simulink model "AUV_Model"  (Simulink 8.2)
settings: Solver=ode4  StartTime=0.0  StopTime=20  FixedStep=0.1  RelTol=1e-3
model workspace (MAT data in the model file):
  cg = Simulink.Signal
  cg.DataType = 'double'
  cg.DocUnits = 'm'
  cg.Dimensions = 3
  cg.DimensionsMode = 'auto'
  cg.Complexity = 'real'
  cg.SampleTime = -1
  cg.SamplingMode = 'Sample based'
  cg.InitialValue = '[0 0 0]'
  m = Simulink.Signal
  m.DataType = 'double'
  m.DocUnits = 'kg'
  m.Dimensions = 1
  m.DimensionsMode = 'auto'
  m.Complexity = 'real'
  m.SampleTime = -1
  m.SamplingMode = 'auto'
  m.InitialValue = '39.00'
  L = Simulink.Signal
  L.DataType = 'double'
  L.DocUnits = 'm'
  L.Dimensions = 1
  L.DimensionsMode = 'auto'
  L.Complexity = 'real'
  L.SampleTime = -1
  L.SamplingMode = 'auto'
  L.InitialValue = '1.065'
  rho = Simulink.Signal
  rho.DataType = 'double'
  rho.DocUnits = 'Kg/m3'
  rho.Dimensions = 1
  rho.DimensionsMode = 'auto'
  rho.Complexity = 'real'
  rho.SampleTime = -1
  rho.SamplingMode = 'auto'
  rho.InitialValue = '1000'
  R = Simulink.Signal
  R.DataType = 'double'
  R.DocUnits = 'm'
  R.Dimensions = 1
  R.DimensionsMode = 'auto'
  R.Complexity = 'real'
  R.SampleTime = -1
  R.SamplingMode = 'auto'
  R.InitialValue = '0.125'
  cb = Simulink.Signal
  cb.DataType = 'double'
  cb.DocUnits = 'm'
  cb.Dimensions = 3
  cb.DimensionsMode = 'auto'
  cb.Complexity = 'real'
  cb.SampleTime = -1
  cb.SamplingMode = 'auto'
  cb.InitialValue = '[0 0 0]'
PostLoadFcn:
  | , if any(exist('dsrtsu_mdlpostloadfcn', 'file') == [2, 3, 6]), try dsrtsu_mdlpostloadfcn('Execute', bdroot); catch fprintf('Error in PostLoadFcn (dsrtsu_mdlpostloadfcn) for model "%s":\n %s\n', bdroot, lasterr); end, end,
InitFcn:
  | b=0;
  | xi=10;
  | yi=10;
  | zi=10;
  | Yawi =0;
  | 
  | x=xi;
  | y=yi;
  | z=zi;
  | yaw=Yawi;
  | pitch=0;
  | roll=0;
  | 
  | xf=20
  | yf=20
  | zf=10
  | %desired time to destination
  | Tdes = 20;
  | 
  | %step count
  | n=Tdes/0.100
StopFcn:
  | % plot3(x,y,-z)
  | plot(x,y)
  |  grid on
  |  axis square
  |  xlabel('x,Surge')
  |  ylabel('y,Sway')
  | % zlabel('-z,Heave')
  |  title('Plot of the AUV path','FontSize',12)
  | % set(p,'Color','red','LineWidth',1)
undefined symbols (not defined in the file): kix, kiy, kpx, kpy
settings Model: DSRTSU_INTERNAL_RTI_VER=360  DSRTSU_INTERNAL_RTI_TYPE=rti1104  Creator=Umesh  LastModifiedBy=Dr. Asokan  ModifiedComment=Umesh -- Fri Jul 22 10:55:36 2011 -- Version 1.4
settings Model: ModifiedHistory=|
  | Umesh -- Fri Jul 22 10:55:36 2011 -- Version 1.4
  | 
  | 
  | Umesh -- Fri Jul 22 10:53:33 2011 -- Version 1.3
  | 
  | 
  | Umesh -- Fri Jul 22 10:49:07 2011 -- Version 1.2
  | 
  | 
  | Umesh -- Fri Jul 22 01:17:32 2011 -- Version 1.1
  | Initial Version of a simple cylindrically shaped AUV
settings OptimizationCC: SimCompilerOptimization=On
settings HardwareCC: ProdIntDivRoundTo=Zero  ProdEndianess=BigEndian  ProdHWDeviceType=Generic->Custom  TargetIntDivRoundTo=Zero  TargetEndianess=BigEndian  TargetHWDeviceType=Generic->Custom
settings SFSimCC: SimParseCustomCode=off
settings RTWCC: SystemTargetFile=rti1104.tlc  MakeCommand=make_rti  TemplateMakefile=rti1104.tmf  Description=dSPACE DS1104 Hardware Platform  ProcessScript=rti1104_make_rtw_hook
settings STFCustomTargetCC: CodeReplacementLibrary=ANSI_C  ParMdlRefBuildCompliant=on  GeneratePreprocessorConditionals=Disable all  SystemTargetFile=rti1104.tlc
settings GRTTargetCC: CompOptLevelCompliant=off  ConcurrentExecutionCompliant=off  MatFileLogging=off  ExtModeMexFile=noextcomm
settings CustomProperty: DataType=RTWOptions_EnumType_F__Installed_Soft_dSPACE_6P6_matlab_rti1104_tlc_rti1104_1InitialSimState  Value=RUN
settings EnumStrPairs: String=RUN

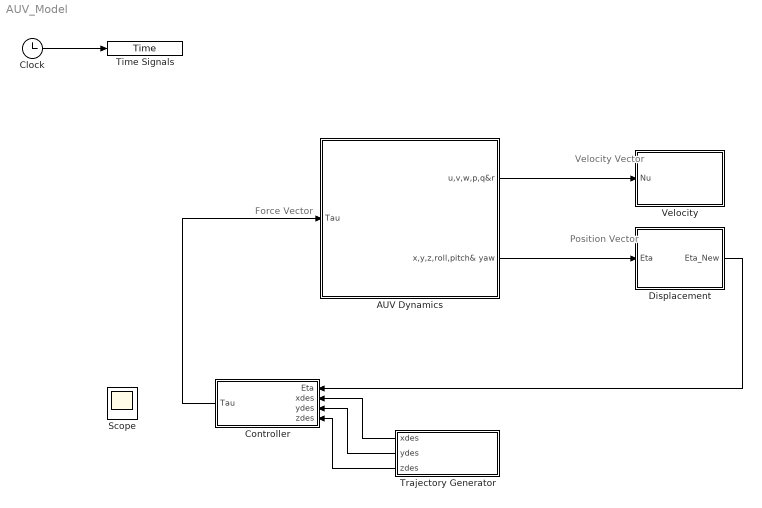
== system AUV_Model ==
  note: Position Vector
  note: Velocity Vector
  note: Force Vector
  AUV Dynamics : Subsystem  Description=Modelled Dynamics of Jubilee AUV, developed by Robotics Lab, IIT Madras
      mask Display: image(imread('Jubilee.jpg'))
  Clock : Clock
  Controller : Subsystem
  Displacement : Subsystem
  Scope : Scope
  Time Signals : ToWorkspace  VariableName=Time  SampleTime=-1
  Trajectory Generator : Subsystem
  Velocity : Subsystem
  wires:
  Clock/1 -> Time Signals/1
  AUV Dynamics/2(x,y,z,roll,pitch& yaw) -> Displacement/1(Eta)
  AUV Dynamics/1(u,v,w,p,q&r) -> Velocity/1(Nu)
  Displacement/1(Eta_New) -> Controller/1(Eta)
  Controller/1(Tau) -> AUV Dynamics/1(Tau)
  Trajectory Generator/2(ydes) -> Controller/3(ydes)
  Trajectory Generator/3(zdes) -> Controller/4(zdes)
  Trajectory Generator/1(xdes) -> Controller/2(xdes)

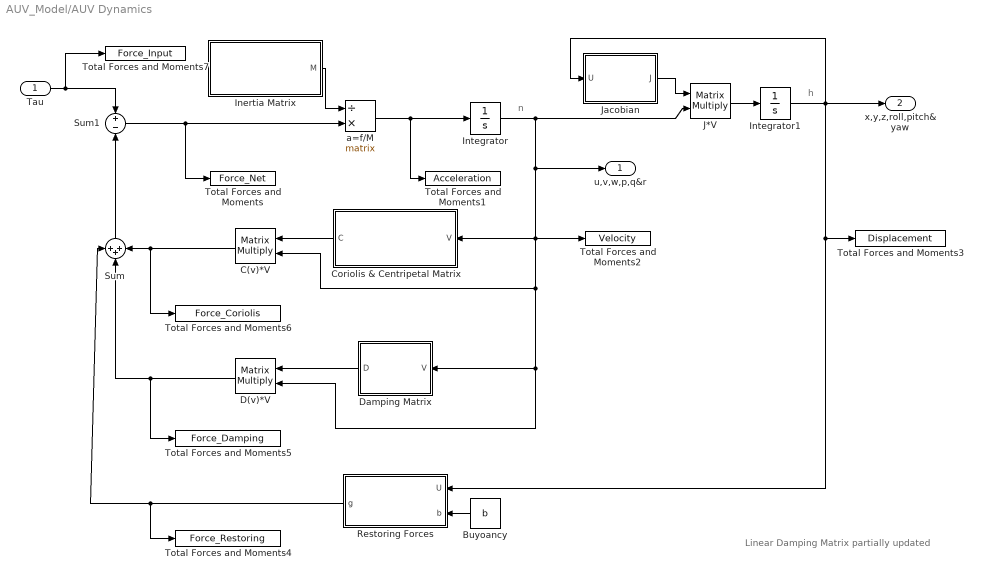
== system AUV_Model/AUV Dynamics ==
  note: h
  note: n
  note: Linear Damping Matrix partially updated
  Tau : Inport
  Buyoancy : Constant  Value=b
  C(v)*V : Product  Inputs=**  Multiplication=Matrix(*)
  Coriolis & Centripetal Matrix : MATLAB Function  TreatAsAtomicUnit=on
  D(v)*V : Product  Inputs=**  Multiplication=Matrix(*)
  Damping Matrix : MATLAB Function  TreatAsAtomicUnit=on
  Inertia Matrix : MATLAB Function  Description=Sub program for Inertia and added mass matrix  TreatAsAtomicUnit=on
  Integrator : Integrator  InitialCondition=[0 0 0 0 0 0]'
  Integrator1 : Integrator  InitialCondition=[xi yi zi 0 0 Yawi*pi/180]'
  J*V : Product  Inputs=**  Multiplication=Matrix(*)
  Jacobian : MATLAB Function  TreatAsAtomicUnit=on
  Restoring Forces : MATLAB Function  TreatAsAtomicUnit=on
  Sum : Sum  Inputs=+++
  Sum1 : Sum  Inputs=+-
  Total Forces and Moments : ToWorkspace  VariableName=Force_Net  SampleTime=-1
  Total Forces and Moments1 : ToWorkspace  VariableName=Acceleration  SampleTime=-1
  Total Forces and Moments2 : ToWorkspace  VariableName=Velocity  SampleTime=-1
  Total Forces and Moments3 : ToWorkspace  VariableName=Displacement  SampleTime=-1
  Total Forces and Moments4 : ToWorkspace  VariableName=Force_Restoring  SampleTime=-1
  Total Forces and Moments5 : ToWorkspace  VariableName=Force_Damping  SampleTime=-1
  Total Forces and Moments6 : ToWorkspace  VariableName=Force_Coriolis  SampleTime=-1
  Total Forces and Moments7 : ToWorkspace  VariableName=Force_Input  SampleTime=-1
  a=f/M : Product  Inputs=/*  Multiplication=Matrix(*)
  u,v,w,p,q&r : Outport
  x,y,z,roll,pitch& yaw : Outport  Port=2
  wires:
  Tau/1 -> Sum1/1, Total Forces and Moments7/1
  Sum1/1 -> Total Forces and Moments/1, a=f/M/2
  a=f/M/1 -> Total Forces and Moments1/1, Integrator/1
  Integrator/1 -> J*V/2, Total Forces and Moments2/1, Coriolis & Centripetal Matrix/1(V), C(v)*V/2, D(v)*V/2, Damping Matrix/1(V), u,v,w,p,q&r/1
  J*V/1 -> Integrator1/1
  Buyoancy/1 -> Restoring Forces/2(b)
  Restoring Forces/1(g) -> Sum/1, Total Forces and Moments4/1
  Sum/1 -> Sum1/2
  D(v)*V/1 -> Sum/2, Total Forces and Moments5/1
  C(v)*V/1 -> Sum/3, Total Forces and Moments6/1
  Integrator1/1 -> x,y,z,roll,pitch& yaw/1, Restoring Forces/1(U), Total Forces and Moments3/1, Jacobian/1(U)
  Jacobian/1(J) -> J*V/1
  Damping Matrix/1(D) -> D(v)*V/1
  Coriolis & Centripetal Matrix/1(C) -> C(v)*V/1
  Inertia Matrix/1(M) -> a=f/M/1

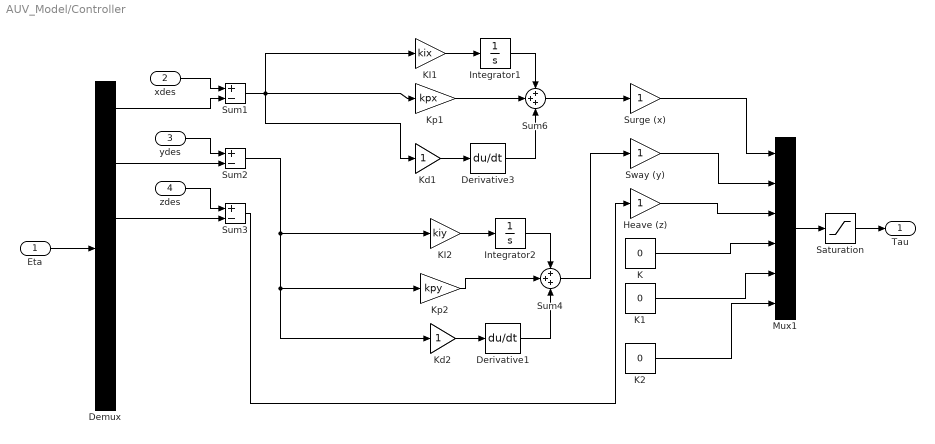
== system AUV_Model/Controller ==
  Eta : Inport
  xdes : Inport  Port=2
  ydes : Inport  Port=3
  zdes : Inport  Port=4
  Demux : Demux  Outputs=6
  Derivative1 : Derivative
  Derivative3 : Derivative
  Heave (z) : Gain
  Integrator1 : Integrator
  Integrator2 : Integrator
  K : Constant  Value=0
  K1 : Constant  Value=0
  K2 : Constant  Value=0
  KI1 : Gain  Gain=kix
  KI2 : Gain  Gain=kiy
  Kd1 : Gain
  Kd2 : Gain
  Kp1 : Gain  Gain=kpx
  Kp2 : Gain  Gain=kpy
  Mux1 : Mux  Inputs=6
  Saturation : Saturate  UpperLimit=56.9  LowerLimit=-56.9
  Sum1 : Sum  Inputs=+-
  Sum2 : Sum  Inputs=+-
  Sum3 : Sum  Inputs=+-
  Sum4 : Sum  Inputs=+++
  Sum6 : Sum  Inputs=+++
  Surge (x) : Gain
  Sway (y) : Gain
  Tau : Outport
  wires:
  Eta/1 -> Demux/1
  xdes/1 -> Sum1/1
  ydes/1 -> Sum2/1
  zdes/1 -> Sum3/1
  Mux1/1 -> Saturation/1
  Sum1/1 -> Kp1/1, KI1/1, Kd1/1
  Sum2/1 -> Kp2/1, Kd2/1, KI2/1
  Sum3/1 -> Heave (z)/1
  Surge (x)/1 -> Mux1/1
  Sway (y)/1 -> Mux1/2
  Heave (z)/1 -> Mux1/3
  K/1 -> Mux1/4
  K1/1 -> Mux1/5
  K2/1 -> Mux1/6
  Saturation/1 -> Tau/1
  Demux/1 -> Sum1/2
  Demux/2 -> Sum2/2
  Demux/3 -> Sum3/2
  Kd1/1 -> Derivative3/1
  KI1/1 -> Integrator1/1
  Integrator1/1 -> Sum6/1
  Derivative3/1 -> Sum6/3
  Kp1/1 -> Sum6/2
  Sum6/1 -> Surge (x)/1
  Kd2/1 -> Derivative1/1
  KI2/1 -> Integrator2/1
  Integrator2/1 -> Sum4/1
  Derivative1/1 -> Sum4/3
  Kp2/1 -> Sum4/2
  Sum4/1 -> Sway (y)/1

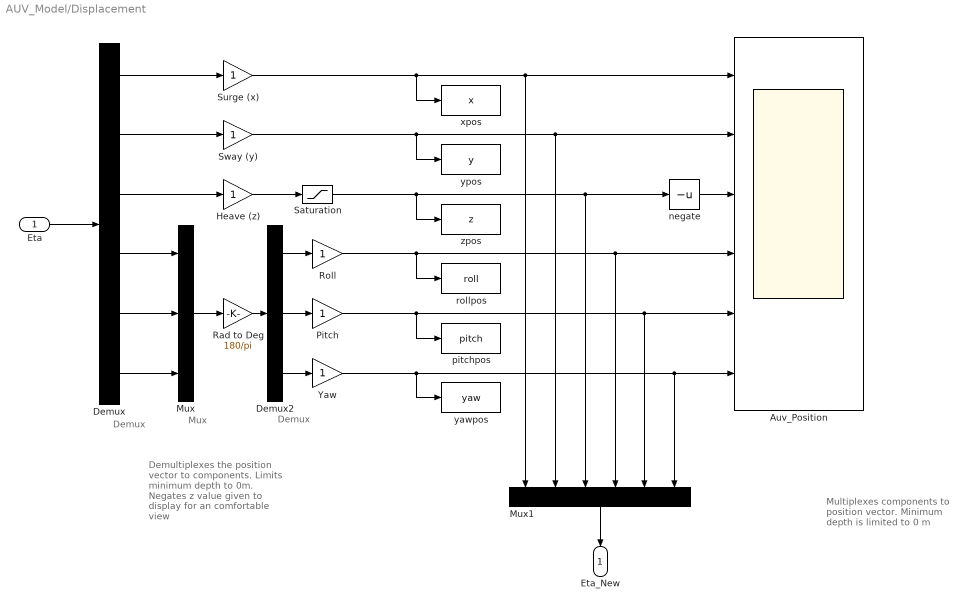
== system AUV_Model/Displacement ==
  note: Demux
  note: Mux
  note: Demux
  note: Demultiplexes the position vector to components.
      | Limits minimum depth to 0m.
      | Negates z value given to display for an comfortable view
  note: Multiplexes components to position vector.
      | Minimum depth is limited to 0 m
  Eta : Inport
  Auv_Position : Scope  NumInputPorts=6
      settings: TickLabels=on  YMin=-50~-1~-25~-1~0~-1  YMax=0~1~-0~1~4~1  SaveName=ScopeData24  MaxDataPoints=10000
  Demux : Demux  Outputs=6
  Demux2 : Demux  Outputs=3
  Heave (z) : Gain
  Mux : Mux  Inputs=3
  Mux1 : Mux  Inputs=6
  Pitch : Gain
  Rad to Deg : Gain  Gain=180/pi
  Roll : Gain
  Saturation : Saturate  UpperLimit=inf  LowerLimit=0
  Surge (x) : Gain
  Sway (y) : Gain
  Yaw : Gain
  negate : UnaryMinus
  pitchpos : ToWorkspace  VariableName=pitch  SampleTime=-1
  rollpos : ToWorkspace  VariableName=roll  SampleTime=-1
  xpos : ToWorkspace  VariableName=x  SampleTime=-1
  yawpos : ToWorkspace  VariableName=yaw  SampleTime=-1
  ypos : ToWorkspace  VariableName=y  SampleTime=-1
  zpos : ToWorkspace  VariableName=z  SampleTime=-1
  Eta_New : Outport
  wires:
  Demux2/3 -> Yaw/1
  Demux2/2 -> Pitch/1
  Demux2/1 -> Roll/1
  Demux/3 -> Heave (z)/1
  Demux/2 -> Sway (y)/1
  Demux/1 -> Surge (x)/1
  Rad to Deg/1 -> Demux2/1
  Mux/1 -> Rad to Deg/1
  Demux/4 -> Mux/1
  Demux/6 -> Mux/3
  Demux/5 -> Mux/2
  Eta/1 -> Demux/1
  Surge (x)/1 -> xpos/1, Auv_Position/1, Mux1/1
  Sway (y)/1 -> ypos/1, Auv_Position/2, Mux1/2
  Heave (z)/1 -> Saturation/1
  negate/1 -> Auv_Position/3
  Saturation/1 -> zpos/1, negate/1, Mux1/3
  Roll/1 -> rollpos/1, Auv_Position/4, Mux1/4
  Pitch/1 -> pitchpos/1, Auv_Position/5, Mux1/5
  Yaw/1 -> yawpos/1, Auv_Position/6, Mux1/6
  Mux1/1 -> Eta_New/1

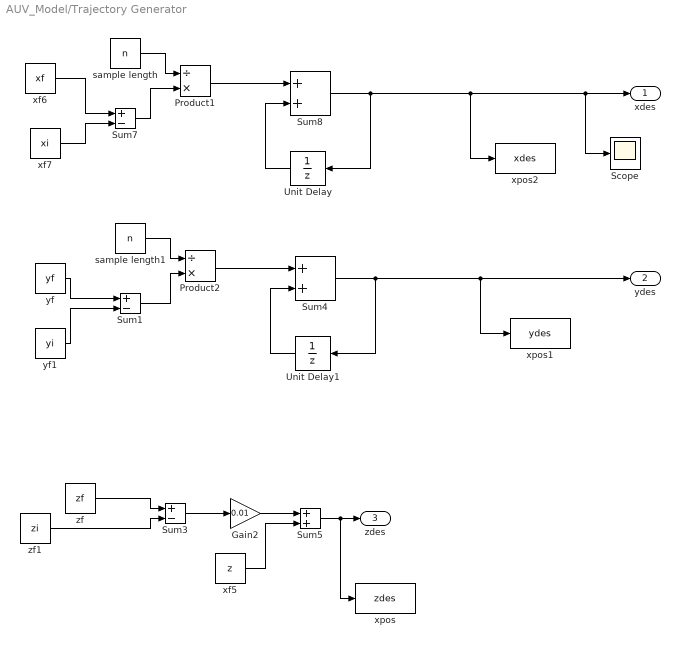
== system AUV_Model/Trajectory Generator ==
  Gain2 : Gain  Gain=0.01
  Product1 : Product  Inputs=/*  RndMeth=Zero
  Product2 : Product  Inputs=/*  RndMeth=Zero
  Scope : Scope
  Sum1 : Sum  Inputs=+-
  Sum3 : Sum  Inputs=+-
  Sum4 : Sum
  Sum5 : Sum
  Sum7 : Sum  Inputs=+-
  Sum8 : Sum
  Unit Delay : UnitDelay  SampleTime=-1
  Unit Delay1 : UnitDelay  SampleTime=-1
  sample length : Constant  Value=n
  sample length1 : Constant  Value=n
  xf5 : Constant  Value=z
  xf6 : Constant  Value=xf
  xf7 : Constant  Value=xi
  xpos : ToWorkspace  VariableName=zdes  SampleTime=-1
  xpos1 : ToWorkspace  VariableName=ydes  SampleTime=-1
  xpos2 : ToWorkspace  VariableName=xdes  SampleTime=-1
  yf : Constant  Value=yf
  yf1 : Constant  Value=yi
  zf : Constant  Value=zf
  zf1 : Constant  Value=zi
  xdes : Outport
  ydes : Outport  Port=2
  zdes : Outport  Port=3
  wires:
  zf1/1 -> Sum3/2
  zf/1 -> Sum3/1
  Sum3/1 -> Gain2/1
  Gain2/1 -> Sum5/1
  Sum5/1 -> zdes/1, xpos/1
  xf5/1 -> Sum5/2
  xf7/1 -> Sum7/2
  xf6/1 -> Sum7/1
  Sum7/1 -> Product1/2
  sample length/1 -> Product1/1
  Product1/1 -> Sum8/1
  Sum8/1 -> Unit Delay/1, Scope/1, xdes/1, xpos2/1
  Unit Delay/1 -> Sum8/2
  Sum1/1 -> Product2/2
  sample length1/1 -> Product2/1
  Product2/1 -> Sum4/1
  Sum4/1 -> Unit Delay1/1, ydes/1, xpos1/1
  Unit Delay1/1 -> Sum4/2
  yf1/1 -> Sum1/2
  yf/1 -> Sum1/1

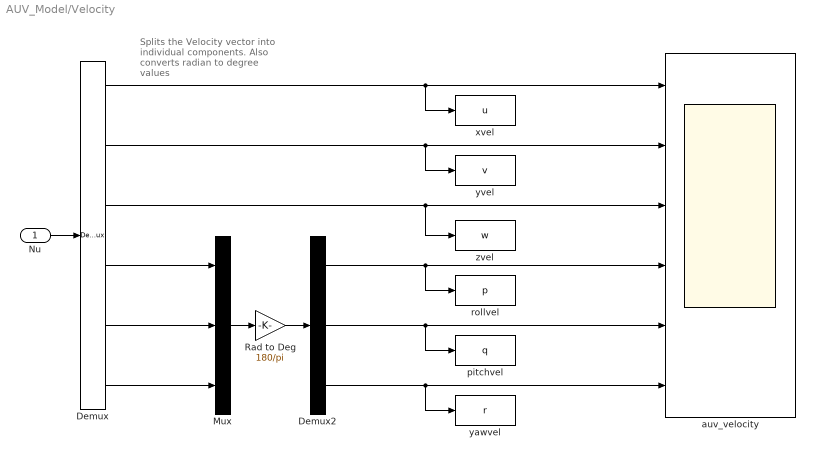
== system AUV_Model/Velocity ==
  note: Splits the Velocity vector into individual components.
      | Also converts radian to degree values
  Nu : Inport
  Demux : Demux  Outputs=6
  Demux2 : Demux  Outputs=3
  Mux : Mux  Inputs=3
  Rad to Deg : Gain  Gain=180/pi
  auv_velocity : Scope  NumInputPorts=6
      settings: TickLabels=on  YMin=-5~-5~-5~-5~-5~-5  YMax=5~5~5~5~5~5  SaveName=ScopeData23  MaxDataPoints=10000
  pitchvel : ToWorkspace  VariableName=q  SampleTime=-1
  rollvel : ToWorkspace  VariableName=p  SampleTime=-1
  xvel : ToWorkspace  VariableName=u  SampleTime=-1
  yawvel : ToWorkspace  VariableName=r  SampleTime=-1
  yvel : ToWorkspace  VariableName=v  SampleTime=-1
  zvel : ToWorkspace  VariableName=w  SampleTime=-1
  wires:
  Demux/5 -> Mux/2
  Demux/6 -> Mux/3
  Mux/1 -> Rad to Deg/1
  Rad to Deg/1 -> Demux2/1
  Nu/1 -> Demux/1
  Demux/4 -> Mux/1
  Demux/1 -> auv_velocity/1, xvel/1
  Demux/2 -> auv_velocity/2, yvel/1
  Demux/3 -> auv_velocity/3, zvel/1
  Demux2/1 -> auv_velocity/4, rollvel/1
  Demux2/2 -> auv_velocity/5, pitchvel/1
  Demux2/3 -> auv_velocity/6, yawvel/1

== matlab function AUV Dynamics/Jacobian ==
  data: U input double; J output double
%-------------------------------------------------------------------------%
%Sub program for computing Jacobian transforming the velocities from body to inertial
%
%Values and calculations for Jubilee AUV, 
%developed by Robotics Lab, Department of Engineering Design, IIT Madras
%
%Code modified on 22/07/2011
%By Umesh Neettiyath
%-------------------------------------------------------------------------%
function J = Jacobian(U)

J1=[cos(U(6))*cos(U(5)) -(sin(U(6))*cos(U(4)))+(cos(U(6))*sin(U(5))*sin(U(4))) (sin(U(6))*sin(U(4)))+(cos(U(6))*cos(U(4))*sin(U(5)));...
    sin(U(6))*cos(U(5)) (cos(U(6))*cos(U(4)))+(sin(U(6))*sin(U(5))*sin(U(4))) -(cos(U(6))*sin(U(4)))+(sin(U(6))*cos(U(4))*sin(U(5)));...
    -sin(U(5)) cos(U(5))*sin(U(4)) cos(U(5))*cos(U(4))];
J2=[1 sin(U(4))*tan(U(5)) cos(U(4))*tan(U(5));...
    0 cos(U(4)) -sin(U(4));...
    0 sin(U(4))/cos(U(5)) cos(U(4))/cos(U(5))];

%Jacobian
J=[J1 zeros(3,3);zeros(3,3) J2];

== matlab function AUV Dynamics/Inertia Matrix ==
  data: M output double; cg data_store_memory double; m data_store_memory double; rho data_store_memory double; L data_store_memory double; R data_store_memory double
%-------------------------------------------------------------------------%
%Sub program for Inertia and added mass matrix  
%
%Values and calculations for Jubilee AUV, 
%developed by Robotics Lab, Department of Engineering Design, IIT Madras
%
%Code modified on 22/07/2011
%By Umesh Neettiyath
%-------------------------------------------------------------------------%
%Use model explorer to modify global variables
%-------------------------------------------------------------------------%
function M = Inertia() % Inertia and Added Mass matrix

global cg; %Centre of gravity
global m;%mass of the vehicle
global L;%vehicle length
global rho;%water density
global R;%Radius of the vehicle

%Centre of gravity
xg=cg(1);yg=cg(2);zg=cg(3);%Centre of gravity

%Inertia values
ixy=0;iyx=ixy;ixz=0;izx=ixz;iyz=0;izy=iyz;
ix=0.34;iy=3.7;iz=3.7;

% Hydrodynamic derivatives
Xudot=-1.170; Xvdot=0; Xwdot=0; Xpdot=0; Xqdot=0; Xrdot=0;
Yudot=0; Yvdot=-34.834; Ywdot=0; Ypdot=0; Yqdot=0; Yrdot=1.042;
Zudot=0; Zvdot=0; Zwdot=-34.834; Zpdot=0; Zqdot=-1.042; Zrdot=0;
Kudot=0; Kvdot=0; Kwdot=0; Kpdot=0; Kqdot=0; Krdot=0;
Mudot=0; Mvdot=0; Mwdot=-1.042; Mpdot=0; Mqdot=-2.659; Mrdot=0; 
Nudot=0; Nvdot=-1.042; Nwdot=0; Npdot=0; Nqdot=0; Nrdot=-2.659;

% Inertia Matrix of Rigid body
Mrb=[m 0 0 0 m*zg -m*yg;...
    0 m 0 -m*zg 0 m*xg;...
    0 0 m m*yg -m*xg 0;...
    0 -m*zg m*yg ix -ixy -ixz;...
    m*zg 0 -m*xg -iyx iy -iyz;...
    -m*yg m*xg 0 -izx -izy iz]; 

% Added Mass matrix
Ma=-[Xudot Xvdot Xwdot Xpdot Xqdot Xrdot;...
    Yudot Yvdot Ywdot Ypdot Yqdot Yrdot;...
    Zudot Zvdot Zwdot Zpdot Zqdot Zrdot;...
    Kudot Kvdot Kwdot Kpdot Kqdot Krdot;...
    Mudot Mvdot Mwdot Mpdot Mqdot Mrdot;...
    Nudot Nvdot Nwdot Npdot Nqdot Nrdot];

% %Total Inertia and mass matrix
M=Mrb+Ma;
%vdot =M\f; %acceleration = inverse(M)*Total force

== matlab function AUV Dynamics/Restoring Forces ==
  data: U input double; g output double; b input double; cb data_store_memory double; cg data_store_memory double; m data_store_memory double
%-------------------------------------------------------------------------%
%Sub program for Restoring effects and its Matrix
%
%Values and calculations for Jubilee AUV, 
%developed by Robotics Lab, Department of Engineering Design, IIT Madras
%
%Code modified on 22/07/2011
%By Umesh Neettiyath
%-------------------------------------------------------------------------%
%Use model explorer to modify global variables
%-------------------------------------------------------------------------%
function g = Restoring_Force(U,b)

global cb; %Centre of buyoancy
global cg; %Centre of gravity
global m;%mass of the vehicle

xg=cg(1);yg=cg(2);zg=cg(3);%Centre of gravity
xb=cb(1);yb=cb(2);zb=cb(3); % Centre of Buoyancy
W=m*9.81;B=(m+b)*9.81;

% Restoring efforts
g=[(W-B)*sin(U(5));...
    -(W-B)*cos(U(5))*sin(U(4));...
    -(W-B)*cos(U(5))*cos(U(4));...
    -(yg*W-yb*B)*cos(U(5))*cos(U(4))+(zg*W-zb*B)*cos(U(5))*sin(U(4));...
  (zg*W-zb*B)*sin(U(5))+(xg*W-xb*B)*cos(U(5))*cos(U(4));...
    -(xg*W-xb*B)*cos(U(5))*sin(U(4))-(yg*W-yb*B)*sin(U(5))];

== matlab function AUV Dynamics/Damping Matrix ==
  data: D output double; V input double; L data_store_memory double; rho data_store_memory double
%-------------------------------------------------------------------------%
%Sub program for calculating the Damping Matrix
%
%Values and calculations for Jubilee AUV, 
%developed by Robotics Lab, Department of Engineering Design, IIT Madras
%
%Code modified on 22/07/2011
%By Umesh Neettiyath
%-------------------------------------------------------------------------%
%Use model explorer to modify global variables
%-------------------------------------------------------------------------%

function D = Damping(V) % Damping Matrix

%Vehicle details
global L;%vehicle length
global rho;%water density

%Vehicle Speed
U = sqrt(V(1)^2+V(2)^2+V(3)^2);

%Hydrodynamic derivative details --to be modified for jubilee
Xu=-2.12; Xv=0; Xw=0; Xp=0; Xq=0; Xr=0;
Yu=0; Yv=-62.45; Yw=0; Yp=0; Yq=0; Yr=0.12;
Zu=0; Zv=0; Zw=-0.1749; Zp=0;  Zr=0;Zq=-0.066873;
Ku=0; Kv=0; Kw=0; Kp=0; Kq=0; Kr=0;
Mu=0; Mv=0;  Mp=0;  Mr=0;Mw=0;Mq=0;
Nu=0; Nv=1.2; Nw=0; Np=0; Nq=0; Nr=-31.25;
%jubilee parameters
Xuu=-7.365;Xvv=0;Xww=-0.737;Xpp=0;Xqq=-1.065;Xrr=-1.065;
Yuu=0;Yvv=-112.2;Yww=0;Ypp=0;Yqq=0;Yrr=0.250;
Zuu=0;Zvv=0;Zww=-112.2;Zpp=0;Zqq=-0.250;Zrr=0;
Kuu=0;Kvv=0;Kww=0;Kpp=0;Kqq=0;Krr=0;
Muu=0;Mvv=0;Mww=2.244;Mpp=0;Mqq=-119.5;Mrr=0;
Nuu=0;Nvv=-2.244;Nww=0;Npp=0;Nqq=0;Nrr=-59.75;

% Linear Damping Matrix
Dvl=-[Xu Xv Xw Xp Xq Xr;...
    Yu Yv Yw Yp Yq Yr;...
    Zu Zv Zw Zp Zq Zr;...
    Ku Kv Kw Kp Kq  Kr ;...
    Mu Mv Mw Mp  Mq  Mr ;...
    Nu Nv Nw Np  Nq  Nr ];

% Quadratic Damping Matrix
Dvq = -[Xuu Xvv Xww Xpp Xqq Xrr;...
    Yuu Yvv Yww Ypp Yqq Yrr;...
    Zuu Zvv Zww Zpp Zqq Zrr;...
    Kuu Kvv Kww Kpp Kqq Krr;...
    Muu Mvv Mww Mpp Mqq Mrr;...
    Nuu Nvv Nww Npp Nqq Nrr];

D = Dvl + Dvq;

== matlab function AUV Dynamics/Coriolis & Centripetal Matrix ==
  data: V input double; C output double; cg data_store_memory double; m data_store_memory double; L data_store_memory double; R data_store_memory double; rho data_store_memory double
%-------------------------------------------------------------------------%
%Sub program for calculating the Coriolis & Centripetal Matrix
%
%Values and calculations for Jubilee AUV, 
%developed by Robotics Lab, Department of Engineering Design, IIT Madras
%
%Code modified on 22/07/2011
%By Umesh Neettiyath
%-------------------------------------------------------------------------%
%Use model explorer to modify global variables
%-------------------------------------------------------------------------%

function C = Coriolis_Centripetal(V) % Coriolis & Centripetal Matrix

global cg; %Centre of gravity
global m;%mass of the vehicle
global L;%vehicle length
global rho;%water density
global R;%Radius of the vehicle

%Centre of gravity
xg=cg(1);yg=cg(2);zg=cg(3);%Centre of gravity

%Inertia values
ixy=0;iyx=ixy;ixz=0;izx=ixz;iyz=0;izy=iyz;
ix=0.34;iy=3.7;iz=3.7;

% Hydrodynamic derivatives
Xudot=-1.170; Xvdot=0; Xwdot=0; Xpdot=0; Xqdot=0; Xrdot=0;
Yudot=0; Yvdot=-34.834; Ywdot=0; Ypdot=0; Yqdot=0; Yrdot=1.042;
Zudot=0; Zvdot=0; Zwdot=-34.834; Zpdot=0; Zqdot=-1.042; Zrdot=0;
Kudot=0; Kvdot=0; Kwdot=0; Kpdot=0; Kqdot=0; Krdot=0;
Mudot=0; Mvdot=0; Mwdot=-1.042; Mpdot=0; Mqdot=-2.659; Mrdot=0; 
Nudot=0; Nvdot=-1.042; Nwdot=0; Npdot=0; Nqdot=0; Nrdot=-2.659;

% Coriolis and Centripetal Forces of Rigid body
Cvrb=[0 0 0 m*(yg*V(5)+zg*V(6)) -m*(xg*V(5)-V(3)) -m*(xg*V(6)+V(2));...
      0 0 0 -m*(yg*V(4)+V(3)) m*(zg*V(6)+xg*V(4)) -m*(yg*V(6)-V(1));...
      0 0 0 -m*(zg*V(4)-V(2)) -m*(zg*V(5)+V(1)) m*(xg*V(4)+yg*V(5));...
      -m*(yg*V(5)+zg*V(6)) m*(yg*V(4)+V(3)) m*(zg*V(4)-V(2)) 0 -iyz*V(5)-ixz*V(4)+iz*V(6) iyz*V(6)+ixy*V(4)-iy*V(5);...
      m*(xg*V(5)-V(3)) -m*(zg*V(6)+xg*V(4)) m*(zg*V(5)+V(1)) iyz*V(5)+ixz*V(4)-iz*V(6) 0 -ixz*V(6)-ixy*V(5)+ix*V(4);...
      m*(xg*V(6)+V(2)) m*(yg*V(6)-V(1)) -m*(xg*V(4)+yg*V(5)) -iyz*V(6)-ixy*V(4)+iy*V(5) ixz*V(6)+ixy*V(5)-ix*V(4) 0];

a1 = Xudot*V(1)+Xvdot*V(2)+Xwdot*V(3)+Xpdot*V(4)+Xqdot*V(5)+Xrdot*V(6);
a2 = Yudot*V(1)+Yvdot*V(2)+Ywdot*V(3)+Ypdot*V(4)+Yqdot*V(5)+Yrdot*V(6);
a3 = Zudot*V(1)+Zvdot*V(2)+Zwdot*V(3)+Zpdot*V(4)+Zqdot*V(5)+Zrdot*V(6);
b1 = Kudot*V(1)+Kvdot*V(2)+Kwdot*V(3)+Kpdot*V(4)+Kqdot*V(5)+Krdot*V(6);
b2 = Mudot*V(1)+Mvdot*V(2)+Mwdot*V(3)+Mpdot*V(4)+Mqdot*V(5)+Mrdot*V(6);
b3 = Nudot*V(1)+Nvdot*V(2)+Nwdot*V(3)+Npdot*V(4)+Nqdot*V(5)+Nrdot*V(6);
  
% Coriolis and Centripetal Forces of Added Mass
c1 = [0 -a3 a2;...
    a3 0 -a1;...
    -a2 a1 0];

c2 = [0 -b3 b2;...
    b3 0 -b1;...
    -b2 b1 0];

Ca=[zeros(3,3) c1;c1 c2];

C=Cvrb+Ca;
